simulink model "compareClosedLoop"  (R2019a)
settings: Solver=ode4  StartTime=0.0  StopTime=1000  FixedStep=0.001  RelTol=1e-3
settings Model: Creator=Juan  LastModifiedBy=Juan
settings DataIOCC: SaveOutput=off  SignalLogging=off  DSMLogging=off  SaveTime=off  ReturnWorkspaceOutputs=off

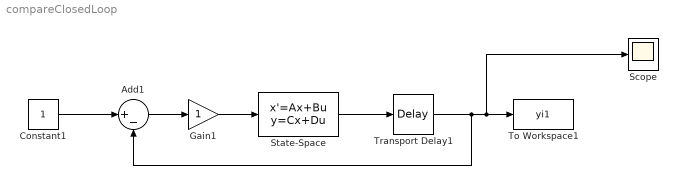
== system compareClosedLoop ==
  Add1 : Sum  Inputs=|+-
  Constant1 : Constant
  Gain1 : Gain
  Scope : Scope
  State-Space : StateSpace  A=[0,-1,-1;1,0.200000000000000,0;2.614035837813944,0,-5.177179722467364]  B=[0;0;0.013333333333333]  C=[0 0 1]  D=0  InitialCondition=[0 0 0]
  To Workspace1 : ToWorkspace  VariableName=yi1  SampleTime=-1
  Transport Delay1 : TransportDelay  DelayTime=300
  wires:
  Add1/1 -> Gain1/1
  State-Space/1 -> Transport Delay1/1
  Gain1/1 -> State-Space/1
  Constant1/1 -> Add1/1
  Transport Delay1/1 -> Add1/2, Scope/1, To Workspace1/1
